simulink model "m20p2"  (R2021b)
settings: Solver=ode45  StartTime=1  StopTime=100  FixedStep=0.1  RelTol=1e-3
undefined symbols (not defined in the file): nmax, nmin, seed
settings Model: Creator=tanzc  LastModifiedBy=tanzc
settings DataIOCC: SaveFormat=Array  ReturnWorkspaceOutputs=off

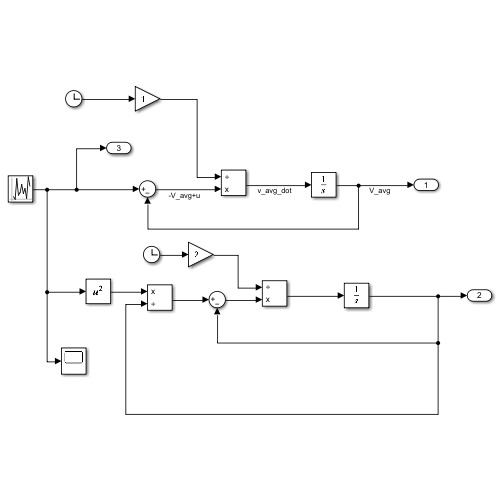
[thumbnail: Simulink's stored preview of the top-level diagram]
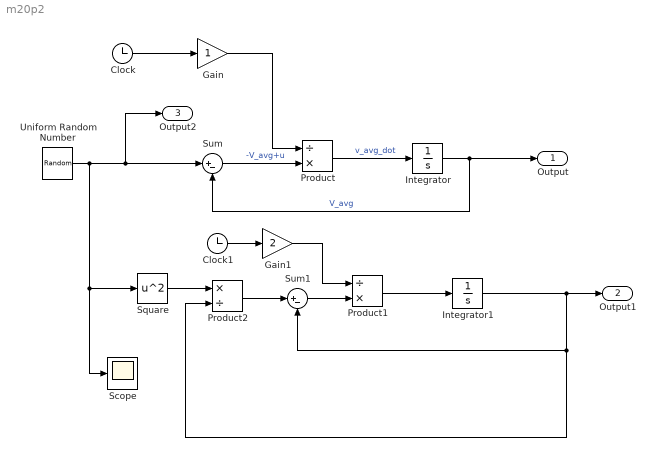
== system m20p2 ==
  Clock : Clock
  Clock1 : Clock
  Gain : Gain
  Gain1 : Gain  Gain=2
  Integrator : Integrator  InitialCondition=0.0001
  Integrator1 : Integrator  InitialCondition=0.0001
  Product : Product  Inputs=/*
  Product1 : Product  Inputs=/*
  Product2 : Product  Inputs=*/
  Scope : Scope
  Square : Math  Operator=square  SaturateOnIntegerOverflow=on
  Sum : Sum  Inputs=|+-
  Sum1 : Sum  Inputs=|+-
  Uniform Random Number : UniformRandomNumber  Minimum=nmin  Maximum=nmax  Seed=seed  SampleTime=1
  Output : Outport
  Output1 : Outport  Port=2
  Output2 : Outport  Port=3
  wires:
  Uniform Random Number/1 -> Scope/1, Square/1, Output2/1, Sum/1
  Integrator/1 -> Output/1, Sum/2  "V_avg"
  Product/1 -> Integrator/1  "v_avg_dot"
  Clock/1 -> Gain/1
  Gain/1 -> Product/1
  Sum/1 -> Product/2  "-V_avg+u"
  Product1/1 -> Integrator1/1
  Clock1/1 -> Gain1/1
  Gain1/1 -> Product1/1
  Square/1 -> Product2/1
  Product2/1 -> Sum1/1
  Integrator1/1 -> Output1/1, Product2/2, Sum1/2
  Sum1/1 -> Product1/2
